simulink model "Hill_sim"  (R2025b)
settings: Solver=VariableStepAuto  StartTime=0.0  StopTime=Tsim  RelTol=1e-3
values from neighbouring files (symbols this model uses):
  m_chaser_kg = 100    [Hill_main.m]
  omega_orb_radps = 0.001259    [Hill_main.m]
  x0_LVLH = [ r0_rel_LVLH_m ... (first row only)    [Hill_main.m]
settings Model: Creator=aayan  LastModifiedBy=aayan

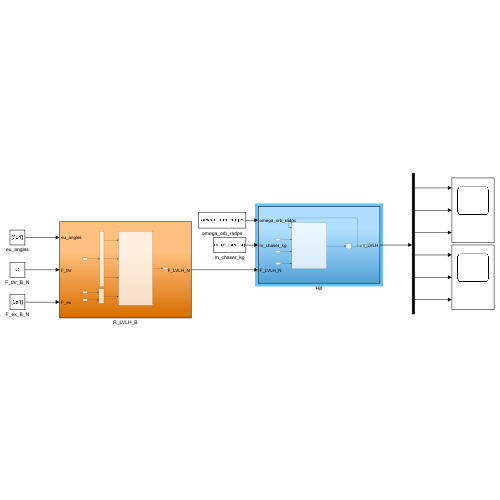
[thumbnail: Simulink's stored preview of the top-level diagram]
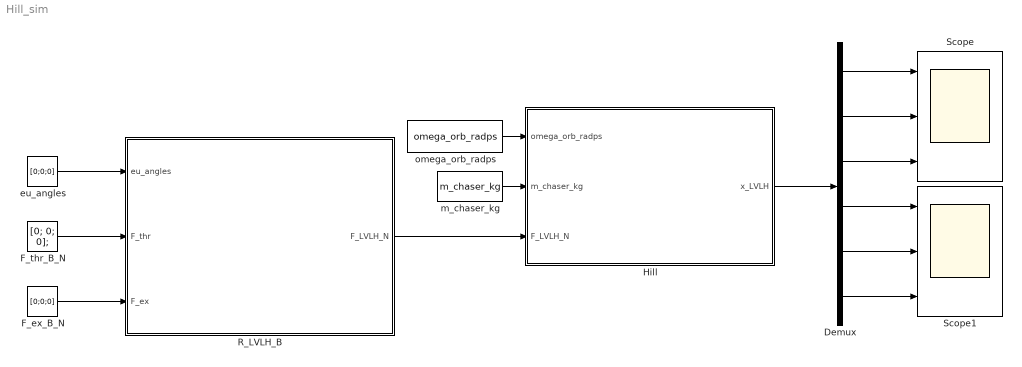
== system Hill_sim ==
  Demux : Demux  Outputs=6
  F_ex_B_N : Constant  Value=[0;0;0]
  F_thr_B_N : Constant  Value=[0; 0; 0];
  Hill : Subsystem
  R_LVLH_B : Subsystem
  Scope : Scope  NumInputPorts=3
      settings: ActiveDisplayYMinimum=20.848112816824809  ActiveDisplayYMaximum=312.36698464857676
  Scope1 : Scope  NumInputPorts=3
      settings: ActiveDisplayYMinimum=-1  ActiveDisplayYMaximum=1
  eu_angles : Constant  Value=[0;0;0]
  m_chaser_kg : Constant  Value=m_chaser_kg
  omega_orb_radps : Constant  Value=omega_orb_radps
  wires:
  F_ex_B_N/1 -> R_LVLH_B/3(F_ex)
  F_thr_B_N/1 -> R_LVLH_B/2(F_thr)
  eu_angles/1 -> R_LVLH_B/1(eu_angles)
  R_LVLH_B/1(F_LVLH_N) -> Hill/3(F_LVLH_N)
  omega_orb_radps/1 -> Hill/1(omega_orb_radps)
  m_chaser_kg/1 -> Hill/2(m_chaser_kg)
  Hill/1(x_LVLH) -> Demux/1
  Demux/1 -> Scope/1
  Demux/2 -> Scope/2
  Demux/3 -> Scope/3
  Demux/4 -> Scope1/1
  Demux/5 -> Scope1/2
  Demux/6 -> Scope1/3

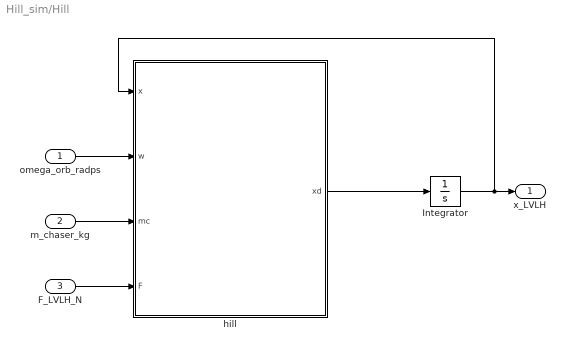
== system Hill_sim/Hill ==
  omega_orb_radps : Inport
  m_chaser_kg : Inport  Port=2
  F_LVLH_N : Inport  Port=3
  Integrator : Integrator  InitialCondition=x0_LVLH
  hill : MATLAB Function  TreatAsAtomicUnit=on
  x_LVLH : Outport
  wires:
  hill/1(xd) -> Integrator/1
  Integrator/1 -> hill/1(x), x_LVLH/1
  F_LVLH_N/1 -> hill/4(F)
  omega_orb_radps/1 -> hill/2(w)
  m_chaser_kg/1 -> hill/3(mc)

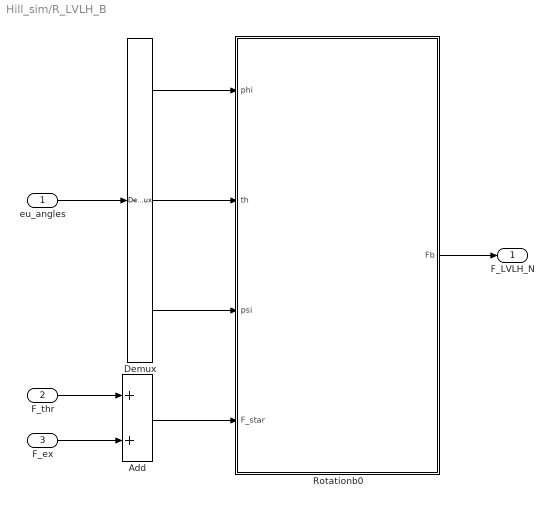
== system Hill_sim/R_LVLH_B ==
  eu_angles : Inport
  F_thr : Inport  Port=2
  F_ex : Inport  Port=3
  Add : Sum
  Demux : Demux  Outputs=3
  Rotationb0 : MATLAB Function  TreatAsAtomicUnit=on
  F_LVLH_N : Outport
  wires:
  F_thr/1 -> Add/1
  F_ex/1 -> Add/2
  Add/1 -> Rotationb0/4(F_star)
  Rotationb0/1(Fb) -> F_LVLH_N/1
  Demux/3 -> Rotationb0/3(psi)
  Demux/2 -> Rotationb0/2(th)
  Demux/1 -> Rotationb0/1(phi)
  eu_angles/1 -> Demux/1

== matlab function Hill_sim/R_LVLH_B/Rotationb0 ==
  data: phi input; th input; psi input; Fb output; F_star input
function Fb = fcn(phi,th,psi,F_star)



Rb0 = eye(3); % To be modified later

Fb = Rb0*F_star

== matlab function Hill_sim/Hill/hill ==
  data: x input; w input; mc input; F input; xd output
function xd = hill(x,w,mc,F)

Fx = F(1);
Fy = F(2);
Fz = F(3);

xd = zeros(6,1);
xd(1:3,1) = x(4:6,1);
xd(4:end,1) = [2*w*x(6) + Fx/mc;         
               -w^2*x(2) + Fy/mc;
               -2*w*x(4) + 3*w^2*x(3) + Fz/mc];
